simulink model "van_der_Pol_typeWalkerModel_Belykh_etal_2017"  (R2022a)
settings: Solver=VariableStepAuto  StartTime=0.0  StopTime=10.0  RelTol=1e-3
settings Model: Creator=Javiera  LastModifiedBy=LEGION
settings SolverCC: AlgebraicLoopSolver=TrustRegion
settings DebuggingCC: UnconnectedInputMsg=warning  UnconnectedOutputMsg=warning  UnconnectedLineMsg=warning  SFMachineParentedDataDiag=warning

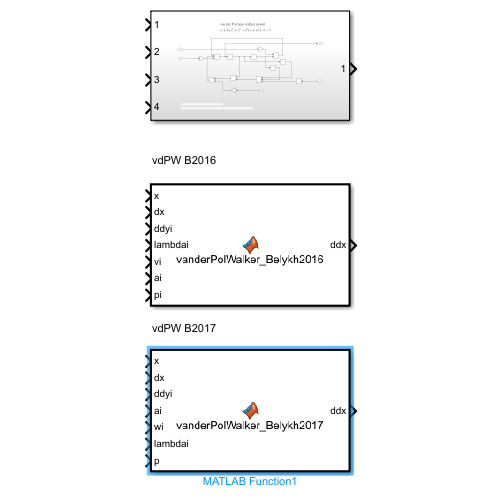
[thumbnail: Simulink's stored preview of the top-level diagram]
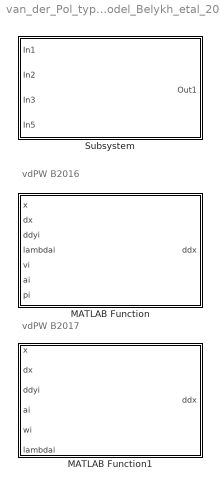
== system van_der_Pol_typeWalkerModel_Belykh_etal_2017 ==
  note: vdPW B2016
  note: vdPW B2017
  MATLAB Function : MATLAB Function  TreatAsAtomicUnit=on
  MATLAB Function1 : MATLAB Function  TreatAsAtomicUnit=on
  Subsystem : Subsystem

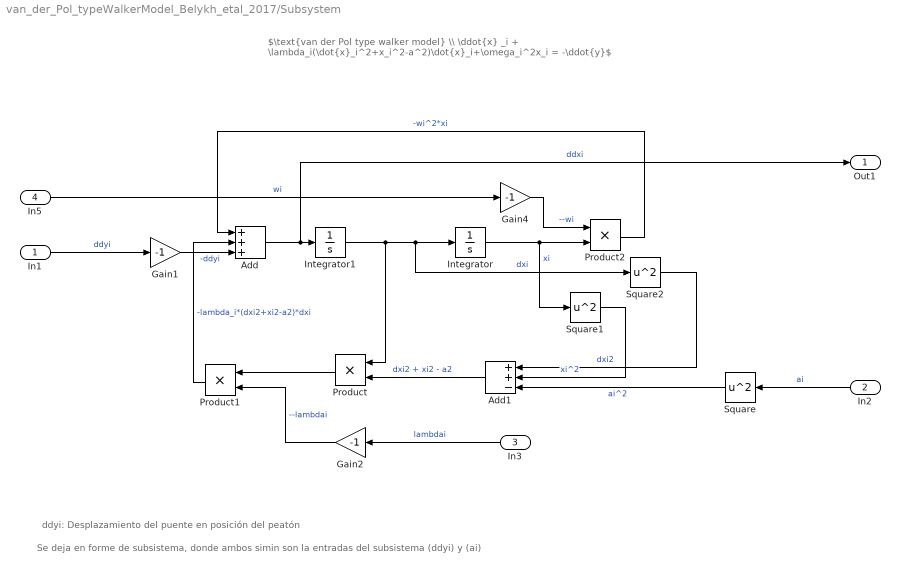
== system van_der_Pol_typeWalkerModel_Belykh_etal_2017/Subsystem ==
  note: ddyi: Desplazamiento del puente en posición del peatón
  note: Se deja en forme de subsistema, donde ambos simin son la entradas del subsistema (ddyi) y (ai)
  note: $\text{van der Pol type walker model} \\ \ddot{x} _i + \lambda_i(\dot{x}_i^2+x_i^2-a^2)\dot{x}_i+\omega_i^2x_i = -\ddot{y}$
  In1 : Inport
  In2 : Inport  Port=2
  In3 : Inport  Port=3
  In5 : Inport  Port=4
  Add : Sum  Inputs=+++
  Add1 : Sum  Inputs=++-
  Gain1 : Gain  Gain=-1
  Gain2 : Gain  Gain=-1
  Gain4 : Gain  Gain=-1
  Integrator : Integrator
  Integrator1 : Integrator
  Product : Product
  Product1 : Product
  Product2 : Product
  Square : Math  Operator=square
  Square1 : Math  Operator=square
  Square2 : Math  Operator=square
  Out1 : Outport
  wires:
  In1/1 -> Gain1/1  "ddyi"
  Integrator1/1 -> Product/1, Square2/1, Integrator/1  "dxi"
  Product1/1 -> Add/2  "-lambda_i*(dxi2+xi2-a2)*dxi"
  Product2/1 -> Add/1  "-wi^2*xi"
  Integrator/1 -> Product2/2, Square1/1  "xi"
  Product/1 -> Product1/1
  Square2/1 -> Add1/1  "dxi2"
  Square/1 -> Add1/3  "ai^2"
  Square1/1 -> Add1/2  "xi^2"
  Add1/1 -> Product/2  "dxi2 + xi2 - a2"
  Gain1/1 -> Add/3  "-ddyi"
  Add/1 -> Out1/1, Integrator1/1  "ddxi"
  In2/1 -> Square/1  "ai"
  Gain2/1 -> Product1/2  "--lambdai"
  In3/1 -> Gain2/1  "lambdai"
  In5/1 -> Gain4/1  "wi"
  Gain4/1 -> Product2/1  "--wi"

== matlab function van_der_Pol_typeWalkerModel_Belykh_etal_2017/MATLAB Function1 ==
  data: x input; ddx output; dx input; ddyi input; ai input; wi input; lambdai input
function ddx = vanderPolWalker_Belykh2017(x,dx,ddyi,ai,wi,lambdai)
% Obtener aceleración del caminante según Belykh et al (2017)
% Alexis Contreras R. 

% Foot force models of crowd dynamics on a wobbly bridge
% Igor V. Belykh, Russel Jeter and Vladimir N. Belykh (2017)

% Modelo de peatón de oscilador auto-sostenible donde los pasos se ajustan
% al movimiento del puente. El balance humano se modela como péndulo invertido.

%%%%%%%%%%%%%%%%%%%%%%%%%%%%%%%%%%%%%%%%%%%%%%%%%%%%%%%%%%%%%%%%%%%%%%%%%%%
% Inputs:
% x         -> Desplazamiento del centro de masa (CoM) del peatón
% dx        -> Velocidad del centro de masa del peatón 
% ddyi      -> Aceleración absoluta del puente (o relativa al suelo/punto fijo externo)
% lambdai   -> Parámetro de amortiguamiento
% ai        -> Parámetro de control del mecanismo de auto-excitación del caminar humano
% wi        -> wi = sqrt(g/L), del modelo pendulo invertido (L >> x)

% Outputs:
% ddx       -> Aceleración del peatón
%%%%%%%%%%%%%%%%%%%%%%%%%%%%%%%%%%%%%%%%%%%%%%%%%%%%%%%%%%%%%%%%%%%%%%%%%%%
% fxdx = lambdai*(dx^2-vi^2*x^2+vi^2*ai^2)*dxi-w0^2*xi; (Eq.4)

fxdx = lambdai*(dx^2+x^2*ai^2)*x + wi^2*x;                                  % (Eq.5)
ddx = -ddyi - fxdx;                                                         % (Eq.1)

== matlab function van_der_Pol_typeWalkerModel_Belykh_etal_2017/MATLAB Function ==
  data: x input; ddx output; dx input; ddyi input; lambdai input; vi input; ai input; pi input
function ddx = vanderPolWalker_Belykh2016(x,dx,ddyi,lambdai,vi,ai,pi)
% Obtener aceleración del caminante según Belykh et al (2016)
% Alexis Contreras R. 

% Bistable gaits and wobbling induced by pedestrian-bridge interactions
% Igor V. Belykh, Russel Jeter and Vladimir N. Belykh (2016)

% Modelo de peatón de oscilador auto-sostenible donde los pasos se ajustan
% al movimiento del puente. El balance humano se modela como péndulo invertido.

%%%%%%%%%%%%%%%%%%%%%%%%%%%%%%%%%%%%%%%%%%%%%%%%%%%%%%%%%%%%%%%%%%%%%%%%%%%
% Inputs:
% x         -> Desplazamiento del centro de masa (CoM) del peatón
% dx        -> Velocidad del centro de masa del peatón 
% ddyi      -> Aceleración absoluta del puente (o relativa al suelo/punto fijo externo)
% lambdai   -> Parámetro de amortiguamiento
% vi        -> Parámetro de control del mecanismo de auto-excitación del caminar humano
% ai        -> Parámetro de control del mecanismo de auto-excitación del caminar humano
% pi        -> Desplazamiento horizontal del centro de presión del pie
% wi        -> wi = sqrt(g/L), del modelo pendulo invertido (L >> x)

% Outputs:
% ddx       -> Aceleración del peatón
%%%%%%%%%%%%%%%%%%%%%%%%%%%%%%%%%%%%%%%%%%%%%%%%%%%%%%%%%%%%%%%%%%%%%%%%%%%

sign_hat = sign(x);                                                         
if x == 0
    sign_hat = 1;                                                           
end

fxdx = lambdai*(dx^2+vi^2*(ai^2-(x-pi*sign_hat)^2))*dx - wi*(x-pi*sign_hat); % (Eq. 2)
ddx = -ddyi - fxdx;                                                         % (Eq. 1)
